simulink model "Modal_observer"  (Simulink 7.7)
settings: Solver=ode45  StartTime=0.0  StopTime=6  RelTol=1e-3
undefined symbols (not defined in the file or in its folder): quad
libraries: simulink x1
settings Model: Creator=Alexey  LastModifiedBy=Alexey

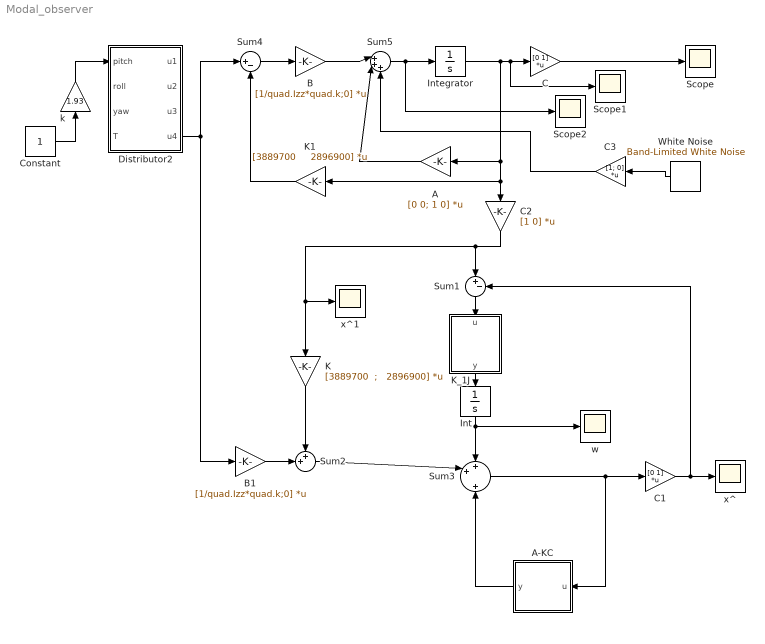
== system Modal_observer ==
  "A " : Gain  Gain=[0 0; 1 0]  Multiplication=Matrix(K*u)
  A-KC : Stateflow chart  TreatAsAtomicUnit=on
  B : Gain  Gain=[1/quad.Izz*quad.k;0]  Multiplication=Matrix(K*u)
  B1 : Gain  Gain=[1/quad.Izz*quad.k;0]  Multiplication=Matrix(K*u)
  C : Gain  Gain=[0 1]  Multiplication=Matrix(K*u)
  C1 : Gain  Gain=[0 1]  Multiplication=Matrix(K*u)
  C2 : Gain  Gain=[1 0]  Multiplication=Matrix(K*u)
  C3 : Gain  Gain=[1; 0]  Multiplication=Matrix(K*u)
  Constant : Constant
  Distributor2 : Subsystem
  Int : Integrator
  Integrator : Integrator
  K : Gain  Gain="[3889700  ;   2896900]"  Multiplication=Matrix(K*u)
  K1 : Gain  Gain="[3889700     2896900]"  Multiplication=Matrix(K*u)
  K_1J : Stateflow chart  TreatAsAtomicUnit=on
  Scope : Scope
      settings: TimeRange=1  YMin=4.195  YMax=4.2325
  Scope1 : Scope
      settings: TimeRange=1  YMin=4.195  YMax=4.2325  SaveName=ScopeData4
  Scope2 : Scope
      settings: TimeRange=1  YMin=4.195  YMax=4.2325  SaveName=ScopeData5
  Sum1 : Sum  Inputs=|+-
  Sum2 : Sum  Inputs=++|
  Sum3 : Sum  Inputs=++|+
  Sum4 : Sum  Inputs=|+-
  Sum5 : Sum  Inputs=|+++
  White Noise : simulink/Sources/Band-Limited White Noise  SystemSampleTime=-1  Cov=[0.001]  Ts=0.01  seed=[233410]
  k : Gain  Gain=1.93
  w : Scope
      settings: TimeRange=1  YMin=-3.4  YMax=-1.2  SaveName=ScopeData2
  x^ : Scope
      settings: TimeRange=1  YMin=0.6  YMax=1.3
  x^1 : Scope
      settings: TimeRange=1  SaveName=ScopeData3
  wires:
  Sum4/1 -> B/1
  B/1 -> Sum5/1
  Sum5/1 -> Integrator/1, Scope2/1
  C/1 -> Scope/1
  "A "/1 -> Sum5/2
  Constant/1 -> k/1
  k/1 -> Distributor2/1(pitch)
  Distributor2/4("u4 ") -> Sum4/1, B1/1
  K/1 -> Sum2/1
  Sum1/1 -> K_1J/1(u)
  Sum2/1 -> Sum3/2
  Sum3/1 -> A-KC/1(u), C1/1
  A-KC/1(y) -> Sum3/3
  K1/1 -> Sum4/2
  K_1J/1(y) -> Int/1
  C3/1 -> Sum5/3
  White Noise/1 -> C3/1
  Int/1 -> w/1, Sum3/1
  C1/1 -> x^/1, Sum1/2
  Integrator/1 -> C/1, Scope1/1, "A "/1, K1/1, C2/1
  B1/1 -> Sum2/2
  C2/1 -> Sum1/1, K/1, x^1/1

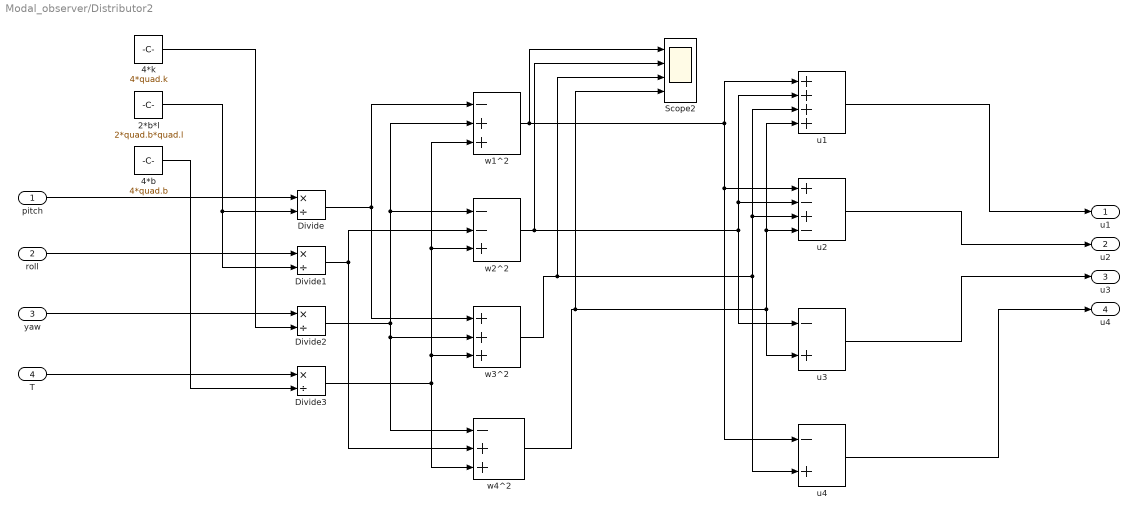
== system Modal_observer/Distributor2 ==
  pitch : Inport
  roll : Inport  Port=2
  yaw : Inport  Port=3
  T : Inport  Port=4
  2*b*l : Constant  Value=2*quad.b*quad.l
  4*b : Constant  Value=4*quad.b
  4*k : Constant  Value=4*quad.k
  Divide{,1..3} (4 alike) : Product  Inputs=*/
  Scope2 : Scope  NumInputPorts=4
      settings: YMin=-1.5e+007~-2.5e+006~-1.5e+007~-2.5e+006  YMax=2.5e+006~1.25e+007~2.5e+006~1.25e+007  SaveName=ScopeData9
  u1 : Sum  Inputs=++++
  u2 : Sum  Inputs=+-+-
  u3 : Sum  Inputs=-+
  u4 : Sum  Inputs=-+
  w1^2 : Sum  Inputs=-++
  w2^2 : Sum  Inputs=--+
  w3^2 : Sum  Inputs=+++
  w4^2 : Sum  Inputs=-++
  "u1 " : Outport
  "u2 " : Outport  Port=2
  "u3 " : Outport  Port=3
  "u4 " : Outport  Port=4
  wires:
  4*k/1 -> Divide2/2
  Divide1/1 -> w4^2/2, w2^2/2
  Divide2/1 -> w3^2/2, w4^2/1, w2^2/1, w1^2/2
  Divide/1 -> w3^2/1, w1^2/1
  4*b/1 -> Divide3/2
  yaw/1 -> Divide2/1
  2*b*l/1 -> Divide/2, Divide1/2
  roll/1 -> Divide1/1
  pitch/1 -> Divide/1
  w1^2/1 -> Scope2/1, u1/1, u2/1, u4/1
  w2^2/1 -> Scope2/2, u1/2, u2/2, u3/1
  w3^2/1 -> Scope2/3, u1/3, u2/3, u4/2
  w4^2/1 -> Scope2/4, u1/4, u2/4, u3/2
  Divide3/1 -> w2^2/3, w1^2/3, w3^2/3, w4^2/3
  T/1 -> Divide3/1
  u1/1 -> "u1 "/1
  u2/1 -> "u2 "/1
  u3/1 -> "u3 "/1
  u4/1 -> "u4 "/1

== matlab function K_1J ==
  data: u input double; y output double
function y = fcn(u)
%#codegen

K1=[0 0; 0 1];
J=[0;1];

y = (K1*J)*u;

== matlab function A-KC ==
  data: u input double; y output double
function y = fcn(u)
%#codegen

A=[0 0; 1 0];
K=[3889700  ;   2896900];
C=[0 1];

y = (A-K*C)*u;
